simulink model "discrete_control_sfunc"  (Simulink 7.4)
settings: Solver=ode45  StartTime=0.0  StopTime=30.0  RelTol=1e-3
values from neighbouring files (symbols this model uses):
  phi0 = 0.15    [discrete_control_angle_from_acc_Driver.m]    (also in discrete_control_sfunc_Driver.m)
  r_psi0 = 0.1    [discrete_control_angle_from_acc_Driver.m]    (also in discrete_control_sfunc_Driver.m)
  theta0 = 0.15    [discrete_control_angle_from_acc_Driver.m]    (also in discrete_control_sfunc_Driver.m)
undefined symbols (not defined in the file or in its folder): boom, DiscIntNeverNeededParam, f1, f2, f3, f4, f5, g, I_x, I_y, I_z, Ts
libraries: Copter_Library x5, simulink x1
CloseFcn:
  | rtwprivate ssgencode ModelCloseRequest discrete_control_sfunc
settings Model: Creator=Robert  LastModifiedBy=roczit00
settings RTWCC: GenCodeOnly=on  GenerateMakefile=off

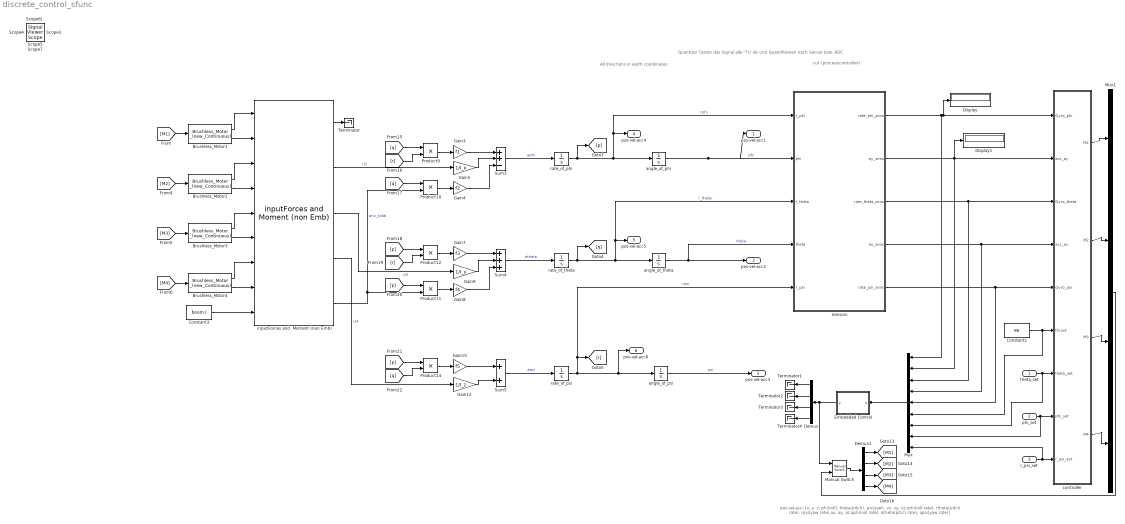
== system discrete_control_sfunc ==
  note: pos-vel-acc: [x, y, z, phi(roll), theta(pitch), psi(yaw), vx, vy, vz,rphi(roll rate), rtheta(pitch rate), rpsi(yaw rate),ax, ay, az,aphi(roll rate), atheta(pitch rate), apsi(yaw rate)]
  note: All directions in earth coordinates
  note: cut (process|controller)
  note: Quantizer Tasten das Signal alle "Ts" ab und Quantifizieren nach Sensor bzw. ADC
  theta_set : Inport  OutDataType=fixdt(1, 16)  OutScaling=2^0
  phi_set : Inport  Port=2  OutDataType=fixdt(1, 16)  OutScaling=2^0
  r_psi_set : Inport  Port=3  OutDataType=fixdt(1, 16)  OutScaling=2^0
  Brushless_Motor{1..4} (4 alike) : Copter_Library/Brushless_Motor _(new_Continuous)  SystemSampleTime=-1  M_error=1
  Constant1 : Constant  Value=90  OutDataType=fixdt(1, 16)  OutScaling=2^0
  Constant3 : Constant  Value=boom.l  OutDataType=fixdt(1, 16)  OutScaling=2^0
  Demux : Demux
  Demux1 : Demux
  Display : Display
  Display1 : Display
  Embedded Control : Stateflow chart
  Gain10 : Gain  Gain=f5  ParameterDataType=fixdt(1, 16)  ParameterScaling=2^0  OutDataType=fixdt(1, 16)  OutScaling=2^0
  Gain12 : Gain  Gain=1/I_z  ParameterDataType=fixdt(1, 16)  ParameterScaling=2^0  OutDataType=fixdt(1, 16)  OutScaling=2^0
  Gain3 : Gain  Gain=f1  ParameterDataType=fixdt(1, 16)  ParameterScaling=2^0  OutDataType=fixdt(1, 16)  OutScaling=2^0
  Gain4 : Gain  Gain=f2  ParameterDataType=fixdt(1, 16)  ParameterScaling=2^0  OutDataType=fixdt(1, 16)  OutScaling=2^0
  Gain5 : Gain  Gain=1/I_x  ParameterDataType=fixdt(1, 16)  ParameterScaling=2^0  OutDataType=fixdt(1, 16)  OutScaling=2^0
  Gain7 : Gain  Gain=f3  ParameterDataType=fixdt(1, 16)  ParameterScaling=2^0  OutDataType=fixdt(1, 16)  OutScaling=2^0
  Gain8 : Gain  Gain=f4  ParameterDataType=fixdt(1, 16)  ParameterScaling=2^0  OutDataType=fixdt(1, 16)  OutScaling=2^0
  Gain9 : Gain  Gain=1/I_y  ParameterDataType=fixdt(1, 16)  ParameterScaling=2^0  OutDataType=fixdt(1, 16)  OutScaling=2^0
  Manual Switch : simulink/Signal Routing/Manual Switch  SystemSampleTime=-1  sw=1  action=0  varsize=off
  Mux : Mux  Inputs=9
  Mux1 : Mux
  Product{9..12,14} (5 alike) : Product  OutDataType=fixdt(1, 16)  OutScaling=2^0  RndMeth=Zero
  Sensors : Subsystem
  Sum3 : Sum  Inputs=++-  OutDataType=fixdt(1, 16)  OutScaling=2^0
  Sum4 : Sum  Inputs=+++  OutDataType=fixdt(1, 16)  OutScaling=2^0
  Sum5 : Sum  OutDataType=fixdt(1, 16)  OutScaling=2^0
  Terminator{,1..4} (5 alike) : Terminator
  angle_of_phi : Integrator  InitialCondition=phi0
  angle_of_psi : Integrator
  angle_of_theta : Integrator  InitialCondition=theta0
  controller : Subsystem
  inputForces and  Moment (non Emb) : Copter_Library/inputForces and  Moment (non Emb)  SystemSampleTime=-1
  rate_of_phi : Integrator
  rate_of_psi : Integrator  InitialCondition=r_psi0
  rate_of_theta : Integrator
  pos-vel-acc1 : Outport  OutDataType=fixdt(1, 16)  OutScaling=2^0
  pos-vel-acc2 : Outport  Port=2  OutDataType=fixdt(1, 16)  OutScaling=2^0
  pos-vel-acc3 : Outport  Port=3  OutDataType=fixdt(1, 16)  OutScaling=2^0
  pos-vel-acc4 : Outport  Port=4  OutDataType=fixdt(1, 16)  OutScaling=2^0
  pos-vel-acc5 : Outport  Port=5  OutDataType=fixdt(1, 16)  OutScaling=2^0
  pos-vel-acc6 : Outport  Port=6  OutDataType=fixdt(1, 16)  OutScaling=2^0
  Scope : SignalViewerScope  IOType=viewer  ZoomMode=yonly  RefreshTime=0.035000
      settings: ShowLegends=on
  Scope1 : SignalViewerScope  IOType=viewer  LegendLocations="214.3333           183            82      20.33333"  RefreshTime=0.035000
      settings: ShowLegends=on
  Scope2 : SignalViewerScope  IOType=viewer  ZoomMode=yonly  RefreshTime=0.035000
      settings: ShowLegends=on  SaveName=ScopeData2
  Scope3 : SignalViewerScope  IOType=viewer  ZoomMode=xonly  RefreshTime=0.035000
      settings: ShowLegends=on  SaveName=ScopeData3
  Scope4 : SignalViewerScope  IOType=viewer  ZoomMode=yonly  RefreshTime=0.035000
      settings: ShowLegends=on  SaveName=ScopeData4
  Scope5 : SignalViewerScope  IOType=viewer  RefreshTime=0.035000
      settings: ShowLegends=on  SaveName=ScopeData5
  Scope6 : SignalViewerScope  IOType=viewer  RefreshTime=0.035000
      settings: ShowLegends=on  SaveName=ScopeData6
  Scope7 : SignalViewerScope  IOType=viewer  LegendLocations="171.2778      154.6944      124.6667         43.25"  RefreshTime=0.035000
      settings: ShowLegends=on  SaveName=ScopeData7
  wires:
  Constant3/1 -> inputForces and  Moment (non Emb)/9
  Sum5/1 -> rate_of_psi/1  "apsi"
  inputForces and  Moment (non Emb)/4 -> Gain12/1  "U4"
  Gain12/1 -> Sum5/2
  Gain10/1 -> Sum5/1
  Product14/1 -> Gain10/1
  [q] -> Product14/2
  [p] -> Product14/1
  Sum4/1 -> rate_of_theta/1  "atheta"
  inputForces and  Moment (non Emb)/3 -> Gain9/1  "U3"
  Gain8/1 -> Sum4/3
  Gain9/1 -> Sum4/2
  Product11/1 -> Gain8/1
  [p] -> Product11/1
  Gain7/1 -> Sum4/1
  Product12/1 -> Gain7/1
  [r] -> Product12/2
  [p] -> Product12/1
  Sum3/1 -> rate_of_phi/1  "aphi"
  Gain4/1 -> Sum3/3
  Gain5/1 -> Sum3/2
  inputForces and  Moment (non Emb)/2 -> Gain5/1  "U2"
  Product10/1 -> Gain4/1
  [q] -> Product10/1
  Gain3/1 -> Sum3/1
  Product9/1 -> Gain3/1
  [r] -> Product9/2
  [q] -> Product9/1
  inputForces and  Moment (non Emb)/5 -> Product11/2, Product10/2  "anv_total"
  angle_of_phi/1 -> pos-vel-acc1/1, Sensors/2(phi)  "phi"
  angle_of_theta/1 -> pos-vel-acc2/1, Sensors/4(theta)  "theta"
  angle_of_psi/1 -> pos-vel-acc3/1  "psi"
  rate_of_phi/1 -> [p], angle_of_phi/1, pos-vel-acc4/1, Sensors/1(r_phi)  "rphi"
  rate_of_theta/1 -> angle_of_theta/1, pos-vel-acc5/1, Sensors/3(r_theta), [q]  "r_theta"
  rate_of_psi/1 -> angle_of_psi/1, pos-vel-acc6/1, [r], Sensors/5(r_psi)  "rpsi"
  Brushless_Motor1/1 -> inputForces and  Moment (non Emb)/1
  Brushless_Motor1/2 -> inputForces and  Moment (non Emb)/2
  Brushless_Motor2/1 -> inputForces and  Moment (non Emb)/3
  Brushless_Motor2/2 -> inputForces and  Moment (non Emb)/4
  Brushless_Motor3/1 -> inputForces and  Moment (non Emb)/5
  Brushless_Motor3/2 -> inputForces and  Moment (non Emb)/6
  Brushless_Motor4/1 -> inputForces and  Moment (non Emb)/7
  Brushless_Motor4/2 -> inputForces and  Moment (non Emb)/8
  inputForces and  Moment (non Emb)/1 -> Terminator/1
  [M1] -> Brushless_Motor1/1
  [M2] -> Brushless_Motor2/1
  [M3] -> Brushless_Motor3/1
  [M4] -> Brushless_Motor4/1
  controller/1(M1) -> Mux1/1
  controller/2(M2) -> Mux1/2
  controller/3(M3) -> Mux1/3
  controller/4(M4) -> Mux1/4
  Constant1/1 -> Mux/6, controller/6(thrust)
  theta_set/1 -> controller/7(theta_set), Mux/7
  phi_set/1 -> controller/8(phi_set), Mux/8
  r_psi_set/1 -> controller/9(r_psi_set), Mux/9
  Sensors/1(rate_phi_sens) -> Mux/1, controller/1(Gyro_phi), Display/1
  Sensors/2(ay_sens) -> controller/2(acc_ay), Mux/2, Display1/1
  Sensors/3(rate_theta_sens) -> controller/3(Gyro_theta), Mux/3
  Sensors/4(ax_sens) -> controller/4(acc_ax), Mux/4
  Sensors/5(rate_psi_sens) -> controller/5(Gyro_psi), Mux/5
  Mux/1 -> Embedded Control/1(u)
  Embedded Control/1(y) -> Demux/1, Manual Switch/1
  Demux/1 -> Terminator1/1
  Demux/2 -> Terminator2/1
  Demux/3 -> Terminator3/1
  Demux/4 -> Terminator4/1
  Manual Switch/1 -> Demux1/1
  Demux1/1 -> [M1]
  Demux1/2 -> [M2]
  Demux1/3 -> [M3]
  Demux1/4 -> [M4]
  Mux1/1 -> Manual Switch/2

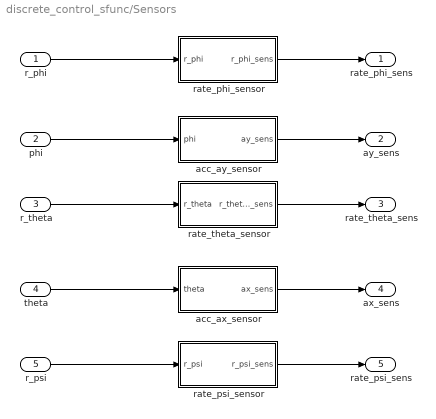
== system discrete_control_sfunc/Sensors ==
  r_phi : Inport  OutDataType=fixdt(1, 16)  OutScaling=2^0
  phi : Inport  Port=2  OutDataType=fixdt(1, 16)  OutScaling=2^0
  r_theta : Inport  Port=3  OutDataType=fixdt(1, 16)  OutScaling=2^0
  theta : Inport  Port=4  OutDataType=fixdt(1, 16)  OutScaling=2^0
  r_psi : Inport  Port=5  OutDataType=fixdt(1, 16)  OutScaling=2^0
  acc_ax_sensor : Subsystem
  acc_ay_sensor : Subsystem
  rate_phi_sensor : Subsystem
  rate_psi_sensor : Subsystem
  rate_theta_sensor : Subsystem
  rate_phi_sens : Outport  OutDataType=fixdt(1, 16)  OutScaling=2^0
  ay_sens : Outport  Port=2  OutDataType=fixdt(1, 16)  OutScaling=2^0
  rate_theta_sens : Outport  Port=3  OutDataType=fixdt(1, 16)  OutScaling=2^0
  ax_sens : Outport  Port=4  OutDataType=fixdt(1, 16)  OutScaling=2^0
  rate_psi_sens : Outport  Port=5  OutDataType=fixdt(1, 16)  OutScaling=2^0
  wires:
  r_phi/1 -> rate_phi_sensor/1(r_phi)
  rate_phi_sensor/1(r_phi_sens) -> rate_phi_sens/1
  phi/1 -> acc_ay_sensor/1(phi)
  acc_ay_sensor/1(ay_sens) -> ay_sens/1
  rate_theta_sensor/1(r_theta_sens) -> rate_theta_sens/1
  acc_ax_sensor/1(ax_sens) -> ax_sens/1
  rate_psi_sensor/1(r_psi_sens) -> rate_psi_sens/1
  r_theta/1 -> rate_theta_sensor/1(r_theta)
  theta/1 -> acc_ax_sensor/1(theta)
  r_psi/1 -> rate_psi_sensor/1(r_psi)

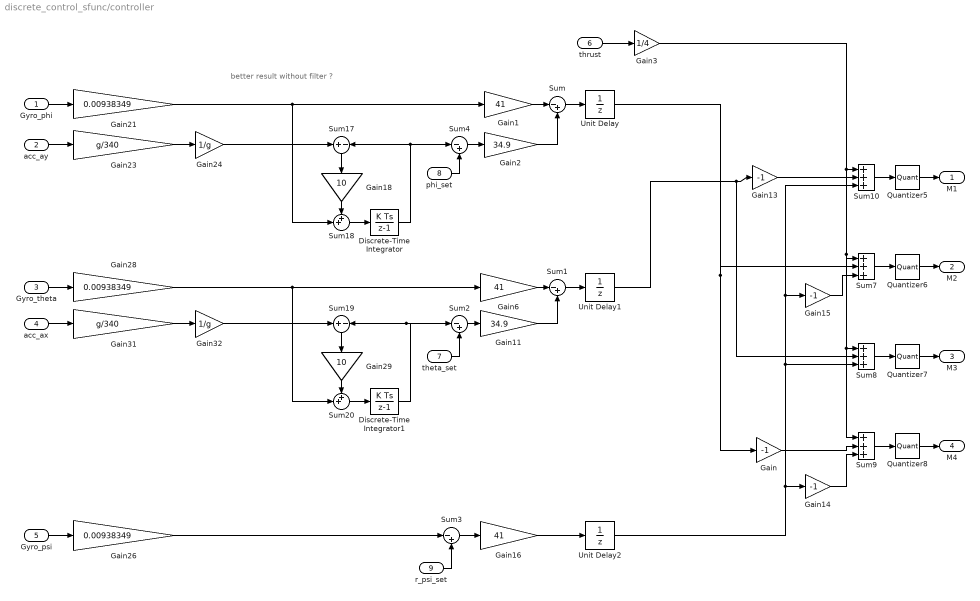
== system discrete_control_sfunc/controller ==
  note: better result without filter ?
  Gyro_phi : Inport  OutDataType=fixdt(1, 16)  OutScaling=2^0
  acc_ay : Inport  Port=2  OutDataType=fixdt(1, 16)  OutScaling=2^0
  Gyro_theta : Inport  Port=3  OutDataType=fixdt(1, 16)  OutScaling=2^0
  acc_ax : Inport  Port=4  OutDataType=fixdt(1, 16)  OutScaling=2^0
  Gyro_psi : Inport  Port=5  OutDataType=fixdt(1, 16)  OutScaling=2^0
  thrust : Inport  Port=6  OutDataType=fixdt(1, 16)  OutScaling=2^0
  theta_set : Inport  Port=7  OutDataType=fixdt(1, 16)  OutScaling=2^0
  phi_set : Inport  Port=8  OutDataType=fixdt(1, 16)  OutScaling=2^0
  r_psi_set : Inport  Port=9  OutDataType=fixdt(1, 16)  OutScaling=2^0
  Discrete-Time Integrator : DiscreteIntegrator  InitialCondition=phi0  SampleTime=Ts  OutDataType=fixdt(1, 16)  OutScaling=2^0  ICPrevOutput=DiscIntNeverNeededParam  ICPrevScaledInput=DiscIntNeverNeededParam
  Discrete-Time Integrator1 : DiscreteIntegrator  InitialCondition=theta0  SampleTime=Ts  OutDataType=fixdt(1, 16)  OutScaling=2^0  ICPrevOutput=DiscIntNeverNeededParam  ICPrevScaledInput=DiscIntNeverNeededParam
  Gain{,13..15} (4 alike) : Gain  Gain=-1  ParameterDataType=fixdt(1, 16)  ParameterScaling=2^0  OutDataType=fixdt(1, 16)  OutScaling=2^0
  Gain1 : Gain  Gain=41  ParameterDataType=fixdt(1, 16)  ParameterScaling=2^0  OutDataType=fixdt(1, 16)  OutScaling=2^0
  Gain11 : Gain  Gain=34.9  ParameterDataType=fixdt(1, 16)  ParameterScaling=2^0  OutDataType=fixdt(1, 16)  OutScaling=2^0
  Gain16 : Gain  Gain=41  ParameterDataType=fixdt(1, 16)  ParameterScaling=2^0  OutDataType=fixdt(1, 16)  OutScaling=2^0
  Gain18 : Gain  Gain=10  ParameterDataType=fixdt(1, 16)  ParameterScaling=2^0  OutDataType=fixdt(1, 16)  OutScaling=2^0
  Gain2 : Gain  Gain=34.9  ParameterDataType=fixdt(1, 16)  ParameterScaling=2^0  OutDataType=fixdt(1, 16)  OutScaling=2^0
  Gain21 : Gain  Gain=0.00938349  ParameterDataType=fixdt(1, 16)  ParameterScaling=2^0  OutDataType=fixdt(1, 16)  OutScaling=2^0
  Gain23 : Gain  Gain=g/340  ParameterDataType=fixdt(1, 16)  ParameterScaling=2^0  OutDataType=fixdt(1, 16)  OutScaling=2^0
  Gain24 : Gain  Gain=1/g  ParameterDataType=fixdt(1, 16)  ParameterScaling=2^0  OutDataType=fixdt(1, 16)  OutScaling=2^0
  Gain26 : Gain  Gain=0.00938349  ParameterDataType=fixdt(1, 16)  ParameterScaling=2^0  OutDataType=fixdt(1, 16)  OutScaling=2^0
  Gain28 : Gain  Gain=0.00938349  ParameterDataType=fixdt(1, 16)  ParameterScaling=2^0  OutDataType=fixdt(1, 16)  OutScaling=2^0
  Gain29 : Gain  Gain=10  ParameterDataType=fixdt(1, 16)  ParameterScaling=2^0  OutDataType=fixdt(1, 16)  OutScaling=2^0
  Gain3 : Gain  Gain=1/4  ParameterDataType=fixdt(1, 16)  ParameterScaling=2^0  OutDataType=fixdt(1, 16)  OutScaling=2^0
  Gain31 : Gain  Gain=g/340  ParameterDataType=fixdt(1, 16)  ParameterScaling=2^0  OutDataType=fixdt(1, 16)  OutScaling=2^0
  Gain32 : Gain  Gain=1/g  ParameterDataType=fixdt(1, 16)  ParameterScaling=2^0  OutDataType=fixdt(1, 16)  OutScaling=2^0
  Gain6 : Gain  Gain=41  ParameterDataType=fixdt(1, 16)  ParameterScaling=2^0  OutDataType=fixdt(1, 16)  OutScaling=2^0
  Quantizer{5..8} (4 alike) : Quantizer  QuantizationInterval=1  SampleTime=Ts
  Sum{,1..4} (5 alike) : Sum  Inputs=|-+  OutDataType=fixdt(1, 16)  OutScaling=2^0
  Sum{7..10} (4 alike) : Sum  Inputs=+++  OutDataType=fixdt(1, 16)  OutScaling=2^0
  Sum17 : Sum  Inputs=+|-  OutDataType=fixdt(1, 16)  OutScaling=2^0
  Sum18 : Sum  Inputs=++|  OutDataType=fixdt(1, 16)  OutScaling=2^0
  Sum19 : Sum  Inputs=+|-  OutDataType=fixdt(1, 16)  OutScaling=2^0
  Sum20 : Sum  Inputs=++|  OutDataType=fixdt(1, 16)  OutScaling=2^0
  Unit Delay : UnitDelay  SampleTime=Ts
  Unit Delay1 : UnitDelay  SampleTime=Ts
  Unit Delay2 : UnitDelay  SampleTime=Ts
  M1 : Outport  OutDataType=fixdt(1, 16)  OutScaling=2^0
  M2 : Outport  Port=2  OutDataType=fixdt(1, 16)  OutScaling=2^0
  M3 : Outport  Port=3  OutDataType=fixdt(1, 16)  OutScaling=2^0
  M4 : Outport  Port=4  OutDataType=fixdt(1, 16)  OutScaling=2^0
  wires:
  Gain1/1 -> Sum/1
  Gain6/1 -> Sum1/1
  Sum/1 -> Unit Delay/1
  Sum1/1 -> Unit Delay1/1
  Unit Delay2/1 -> Gain14/1, Sum8/3, Gain15/1, Sum10/3
  Unit Delay/1 -> Gain/1, Sum7/2
  Unit Delay1/1 -> Gain13/1, Sum8/2
  Gain3/1 -> Sum10/1, Sum7/1, Sum8/1, Sum9/1
  Gain13/1 -> Sum10/2
  Gain/1 -> Sum9/2
  Gain15/1 -> Sum7/3
  Gain14/1 -> Sum9/3
  Sum10/1 -> Quantizer5/1
  Sum7/1 -> Quantizer6/1
  Sum8/1 -> Quantizer7/1
  Sum9/1 -> Quantizer8/1
  Sum18/1 -> Discrete-Time Integrator/1
  Gain18/1 -> Sum18/1
  Sum17/1 -> Gain18/1
  Gain21/1 -> Sum18/2, Gain1/1
  Gain23/1 -> Gain24/1
  Gain24/1 -> Sum17/1
  Gain28/1 -> Sum20/2, Gain6/1
  Sum20/1 -> Discrete-Time Integrator1/1
  Gain29/1 -> Sum20/1
  Sum19/1 -> Gain29/1
  Gain31/1 -> Gain32/1
  Gain32/1 -> Sum19/1
  Discrete-Time Integrator/1 -> Sum17/2, Sum4/1
  Discrete-Time Integrator1/1 -> Sum19/2, Sum2/1
  Quantizer5/1 -> M1/1
  Quantizer6/1 -> M2/1
  Quantizer7/1 -> M3/1
  Quantizer8/1 -> M4/1
  Gyro_psi/1 -> Gain26/1
  acc_ax/1 -> Gain31/1
  Gyro_theta/1 -> Gain28/1
  acc_ay/1 -> Gain23/1
  Gyro_phi/1 -> Gain21/1
  Gain2/1 -> Sum/2
  Gain11/1 -> Sum1/2
  Gain16/1 -> Unit Delay2/1
  Sum4/1 -> Gain2/1
  phi_set/1 -> Sum4/2
  Sum2/1 -> Gain11/1
  theta_set/1 -> Sum2/2
  r_psi_set/1 -> Sum3/2
  Sum3/1 -> Gain16/1
  Gain26/1 -> Sum3/1
  thrust/1 -> Gain3/1

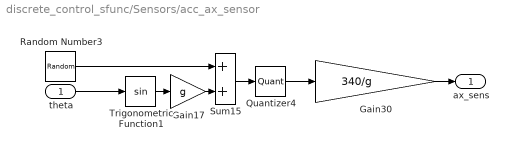
== system discrete_control_sfunc/Sensors/acc_ax_sensor ==
  theta : Inport  OutDataType=fixdt(1, 16)  OutScaling=2^0
  Gain17 : Gain  Gain=g  ParameterDataType=fixdt(1, 16)  ParameterScaling=2^0  OutDataType=fixdt(1, 16)  OutScaling=2^0
  Gain30 : Gain  Gain=340/g  ParameterDataType=fixdt(1, 16)  ParameterScaling=2^0  OutDataType=fixdt(1, 16)  OutScaling=2^0
  Quantizer4 : Quantizer  QuantizationInterval=g/340  SampleTime=Ts
  Random Number3 : RandomNumber  Variance=0.0003  Seed=676  SampleTime=Ts
  Sum15 : Sum  OutDataType=fixdt(1, 16)  OutScaling=2^0
  Trigonometric Function1 : Trigonometry
  ax_sens : Outport  OutDataType=fixdt(1, 16)  OutScaling=2^0
  wires:
  Random Number3/1 -> Sum15/1
  Sum15/1 -> Quantizer4/1
  Trigonometric Function1/1 -> Gain17/1
  Gain17/1 -> Sum15/2
  Quantizer4/1 -> Gain30/1
  theta/1 -> Trigonometric Function1/1
  Gain30/1 -> ax_sens/1

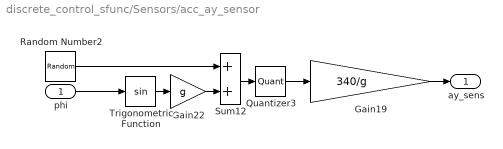
== system discrete_control_sfunc/Sensors/acc_ay_sensor ==
  phi : Inport  OutDataType=fixdt(1, 16)  OutScaling=2^0
  Gain19 : Gain  Gain=340/g  ParameterDataType=fixdt(1, 16)  ParameterScaling=2^0  OutDataType=fixdt(1, 16)  OutScaling=2^0
  Gain22 : Gain  Gain=g  ParameterDataType=fixdt(1, 16)  ParameterScaling=2^0  OutDataType=fixdt(1, 16)  OutScaling=2^0
  Quantizer3 : Quantizer  QuantizationInterval=g/340  SampleTime=Ts
  Random Number2 : RandomNumber  Variance=0.0003  Seed=4564  SampleTime=0.01
  Sum12 : Sum  OutDataType=fixdt(1, 16)  OutScaling=2^0
  Trigonometric Function : Trigonometry
  ay_sens : Outport  OutDataType=fixdt(1, 16)  OutScaling=2^0
  wires:
  Random Number2/1 -> Sum12/1
  Sum12/1 -> Quantizer3/1
  Trigonometric Function/1 -> Gain22/1
  Gain22/1 -> Sum12/2
  Quantizer3/1 -> Gain19/1
  phi/1 -> Trigonometric Function/1
  Gain19/1 -> ay_sens/1

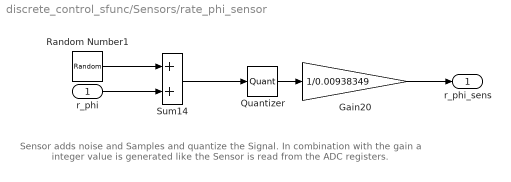
== system discrete_control_sfunc/Sensors/rate_phi_sensor ==
  note: Sensor adds noise and Samples and quantize the Signal. In combination with the gain a integer value is generated
      | like the Sensor is read from the ADC registers.
  r_phi : Inport  OutDataType=fixdt(1, 16)  OutScaling=2^0
  Gain20 : Gain  Gain=1/0.00938349  ParameterDataType=fixdt(1, 16)  ParameterScaling=2^0  OutDataType=fixdt(1, 16)  OutScaling=2^0
  Quantizer : Quantizer  QuantizationInterval=0.00938349  SampleTime=Ts
  Random Number1 : RandomNumber  Variance=3.0462e-8  Seed=45632  SampleTime=0.01
  Sum14 : Sum  OutDataType=fixdt(1, 16)  OutScaling=2^0
  r_phi_sens : Outport  OutDataType=fixdt(1, 16)  OutScaling=2^0
  wires:
  Random Number1/1 -> Sum14/1
  Sum14/1 -> Quantizer/1
  Quantizer/1 -> Gain20/1
  r_phi/1 -> Sum14/2
  Gain20/1 -> r_phi_sens/1

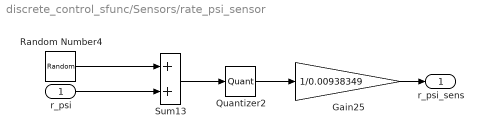
== system discrete_control_sfunc/Sensors/rate_psi_sensor ==
  r_psi : Inport  OutDataType=fixdt(1, 16)  OutScaling=2^0
  Gain25 : Gain  Gain=1/0.00938349  ParameterDataType=fixdt(1, 16)  ParameterScaling=2^0  OutDataType=fixdt(1, 16)  OutScaling=2^0
  Quantizer2 : Quantizer  QuantizationInterval=0.00938349  SampleTime=Ts
  Random Number4 : RandomNumber  Variance=3.0462e-8  Seed=1634  SampleTime=0.01
  Sum13 : Sum  OutDataType=fixdt(1, 16)  OutScaling=2^0
  r_psi_sens : Outport  OutDataType=fixdt(1, 16)  OutScaling=2^0
  wires:
  Random Number4/1 -> Sum13/1
  Sum13/1 -> Quantizer2/1
  Quantizer2/1 -> Gain25/1
  r_psi/1 -> Sum13/2
  Gain25/1 -> r_psi_sens/1

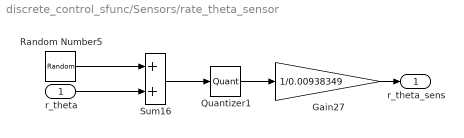
== system discrete_control_sfunc/Sensors/rate_theta_sensor ==
  r_theta : Inport  OutDataType=fixdt(1, 16)  OutScaling=2^0
  Gain27 : Gain  Gain=1/0.00938349  ParameterDataType=fixdt(1, 16)  ParameterScaling=2^0  OutDataType=fixdt(1, 16)  OutScaling=2^0
  Quantizer1 : Quantizer  QuantizationInterval=0.00938349  SampleTime=Ts
  Random Number5 : RandomNumber  Variance=3.0462e-8  Seed=4731  SampleTime=0.01
  Sum16 : Sum  OutDataType=fixdt(1, 16)  OutScaling=2^0
  r_theta_sens : Outport  OutDataType=fixdt(1, 16)  OutScaling=2^0
  wires:
  Random Number5/1 -> Sum16/1
  Sum16/1 -> Quantizer1/1
  Quantizer1/1 -> Gain27/1
  r_theta/1 -> Sum16/2
  Gain27/1 -> r_theta_sens/1

== matlab function Embedded Control ==
  data: u input double; y output double
function y = fcn(u)
%#eml
persistent phi_filt theta_filt M1 M2 M3 M4
%  first time initialization
if isempty(M1) 
    M1=int8(0);
end
if isempty(M2) 
    M2=int8(0);
end
if isempty(M3) 
    M3=int8(0);
end
if isempty(M4) 
    M4=int8(0);
end
if isempty(phi_filt) 
    phi_filt=0.15;
end
if isempty(theta_filt) 
    theta_filt=0.15;
end
Ts = 0.01;
% copy inputs to variables with easy to know names
Gyro_phi =  u(3);
acc_ay = u(2);
Gyro_theta = u(4);
acc_ax = u(4);
Gyro_psi = u(5);
thrust = u(6);
theta_set = u(7);
phi_set = u(8);
r_psi_set = u(9);

% Set outputs to Values calculated last sample time
y = double([M1;M2;M3;M4]);

% Filter berechnen
phi_filt = phi_filt +Ts*((Gyro_phi * 0.00938349) + (acc_ay * (9.81/340)/ 9.81 - phi_filt)*10);
theta_filt = theta_filt +Ts*((Gyro_theta * 0.00938349) + (acc_ax * (9.81/340) / 9.81 - theta_filt)*10);
% e-phi
e_phi=-(Gyro_phi * 0.00938349)*41.0+(phi_set-phi_filt)*34.9;
e_theta=-(Gyro_theta * 0.00938349)*41.0+(theta_set-theta_filt)*34.9;
e_psi=-((Gyro_psi * 0.00938349)-r_psi_set)*41.0;

%neu Ausgabewerte berechnen
M1=int8(thrust/4-e_theta+e_psi);
M2=int8(thrust/4+e_phi-e_psi);
M3=int8(thrust/4+e_theta+e_psi);
M4=int8(thrust/4-e_phi-e_psi);
